simulink model "Dyn_6DoF_v2_0_r2019b"  (R2019b)
settings: Solver=ode4  StartTime=0.0  StopTime=simInit.TSIM  FixedStep=simInit.dt  MaxStep=simInit.dt  RelTol=1e-3
InitFcn:
  | close all
undefined symbols (not defined in the file): __PRM__SERIALIZED__DATA__, act, constr, DE2019, DiscIntNeverNeededParam, ENVMT, omega_rate_max, params, simInit, SubsystemReferenceBlock
libraries: simulink x16, simulink_extras x3
(part 3 of 3)

== matlab function Dyn_6DoF_v2_0_r2019b/AirborneSystem/ForcesAndTorques/aerodynamic forces FSI/Elevator Aero/Elevator_aero ==
  data: input input double; out output double size=[6,1]; DE2019 parameter; ENVMT parameter
% Copyright 2021 Delft University of Technology
%
% Licensed under the Apache License, Version 2.0 (the "License");
% you may not use this file except in compliance with the License.
% You may obtain a copy of the License at
%
%      http://www.apache.org/licenses/LICENSE-2.0
%
% Unless required by applicable law or agreed to in writing, software
% distributed under the License is distributed on an "AS IS" BASIS,
% WITHOUT WARRANTIES OR CONDITIONS OF ANY KIND, either express or implied.
% See the License for the specific language governing permissions and
% limitations under the License.

function out = simpleAero(input, DE2019, ENVMT)
%simpleAero - Elevator simple aero calculation
%
% Inputs:
%    input  - airspeed, AoA, sideslip, CL and CD
%    DE2019 - Aircraft parameters
%    ENVMT  - Environment characteristics
%
% Outputs:
%    out    - 3D forces and moments generated by the elevator
%
%
% Author: Sebastian Rapp, Ph.D., Revised by: Dylan Eijkelhof, M.Sc.
% Delft University of Technology
% email address: d.eijkelhof@tudelft.nl
% December 2019; Last revision: 19-March-2021

%-------------	BEGIN CODE	--------------
    V = input(1);
    alpha = input(2);
    beta = input(3);

    q = 0.5*ENVMT.rhos*V^2;

    F_L_el = -input(4)*q*DE2019.S_el;
    F_D_el = -input(5)*q*DE2019.S_el;

    F_x_s = F_D_el*cos(alpha)*cos(beta) - F_L_el*sin(alpha)*cos(beta);
    F_y_s = 0;
    F_z_s = F_L_el*cos(alpha);

    M_x_s = 0;
    M_y_s = F_L_el*(DE2019.x_el+DE2019.c_el*0.25);
    M_z_s = 0;

    out = [F_x_s, F_y_s, F_z_s, M_x_s, M_y_s, M_z_s]';
%-------------	END CODE	--------------
end

== matlab function Dyn_6DoF_v2_0_r2019b/AirborneSystem/FlightControlSystem/AttitudeAndRateLoop/RateLoop/Rate_Loop/Hedging/InversionRotationalDynamics1 ==
  data: nu_p_hat output; Moments input; p input; q input; r input; DE2019 parameter; nu_q_hat output; nu_r_hat output
% Copyright 2021 Delft University of Technology
%
% Licensed under the Apache License, Version 2.0 (the "License");
% you may not use this file except in compliance with the License.
% You may obtain a copy of the License at
%
%      http://www.apache.org/licenses/LICENSE-2.0
%
% Unless required by applicable law or agreed to in writing, software
% distributed under the License is distributed on an "AS IS" BASIS,
% WITHOUT WARRANTIES OR CONDITIONS OF ANY KIND, either express or implied.
% See the License for the specific language governing permissions and
% limitations under the License.

function [nu_p_hat, nu_q_hat, nu_r_hat] = hedging_rot_inv(Moments, p, q, r, DE2019)
%hedging_rot_inv - Expected error after inversion
%
% Inputs:
%    Moments   - Roll, pitch and yaw moment
%    p         - Roll rate
%    q         - Pitch rate
%    r         - Yaw rate
%    DE2019    - Aircraft parameters
%
% Outputs:
%    nu_p_hat  - Expected roll rate error
%    nu_q_hat  - Expected pitch rate error
%    nu_r_hat  - Expected yaw rate error
%
% Other m-files required:   none
% Subfunctions:             none
% MAT-files required:       none
%
% Author: Sebastian Rapp, Ph.D., Revised by: Dylan Eijkelhof, M.Sc.
% Delft University of Technology
% email address: d.eijkelhof@tudelft.nl
% December 2019; Last revision: 19-March-2021

%------------- BEGIN CODE --------------
 
L = Moments(1); 
M = Moments(2); 
N = Moments(3); 

Jx =  DE2019.J(1,1); 
Jy =  DE2019.J(2,2); 
Jz =  DE2019.J(3,3); 
 
nu_p_hat = 1/Jx * (L - q * r * Jz +  q * r * Jy ); 
nu_q_hat = 1/Jy *(M - r * p * Jx + r * p * Jz  );
nu_r_hat = 1/Jz * (N - p * q * Jy + p * q * Jx ); 

%------------- END CODE --------------
end

== matlab function Dyn_6DoF_v2_0_r2019b/AirborneSystem/FlightControlSystem/AttitudeAndRateLoop/RateLoop/Rate_Loop/InversionRotationalDynamics ==
  data: omega_OB_B input; M_des output; nu_NDI input; DE2019 parameter
% Copyright 2021 Delft University of Technology
%
% Licensed under the Apache License, Version 2.0 (the "License");
% you may not use this file except in compliance with the License.
% You may obtain a copy of the License at
%
%      http://www.apache.org/licenses/LICENSE-2.0
%
% Unless required by applicable law or agreed to in writing, software
% distributed under the License is distributed on an "AS IS" BASIS,
% WITHOUT WARRANTIES OR CONDITIONS OF ANY KIND, either express or implied.
% See the License for the specific language governing permissions and
% limitations under the License.

function M_des  = Rate_inv(omega_OB_B,nu_NDI,  DE2019)
%Rate_inv - Determine desired moments
%
% Inputs:
%    omega_OB_B - Commanded roll, pitch and yaw rates
%    nu_NDI     - Roll, pitch and yaw rate error incl. controller gains
%    DE2019     - Aircraft parameters
%
% Outputs:
%    M_des  - Expected roll rate error
%
% Other m-files required:   none
% Subfunctions:             none
% MAT-files required:       none
%
% Author: Sebastian Rapp, Ph.D., Revised by: Dylan Eijkelhof, M.Sc.
% Delft University of Technology
% email address: d.eijkelhof@tudelft.nl
% December 2019; Last revision: 19-March-2021

%------------- BEGIN CODE --------------

p = omega_OB_B(1); 
q = omega_OB_B(2); 
r = omega_OB_B(3); 

nu_p = nu_NDI(1); 
nu_q = nu_NDI(2); 
nu_r = nu_NDI(3); 
 
Jx = DE2019.J(1,1); 
Jy = DE2019.J(2,2); 
Jz = DE2019.J(3,3);

Lc = Jx * nu_p + q * r * Jz  - q * r * Jy; 
Mc = Jy * nu_q + r * p * Jx - r * p * Jz;
Nc = Jz * nu_r + p * q * Jy - p * q * Jx; 

M_des = [Lc; Mc; Nc];

%------------- END CODE --------------
end

== matlab function Dyn_6DoF_v2_0_r2019b/AirborneSystem/ForcesAndTorques/aerodynamic forces FSI/Rudder Aero/Rudder_aero ==
  data: input input double; out output double size=[6,1]; DE2019 parameter; ENVMT parameter
% Copyright 2021 Delft University of Technology
%
% Licensed under the Apache License, Version 2.0 (the "License");
% you may not use this file except in compliance with the License.
% You may obtain a copy of the License at
%
%      http://www.apache.org/licenses/LICENSE-2.0
%
% Unless required by applicable law or agreed to in writing, software
% distributed under the License is distributed on an "AS IS" BASIS,
% WITHOUT WARRANTIES OR CONDITIONS OF ANY KIND, either express or implied.
% See the License for the specific language governing permissions and
% limitations under the License.

function out = simpleAero(input, DE2019, ENVMT)
%simpleAero - Rudder simple aero calculation
%
% Inputs:
%    input  - airspeed, AoA, sideslip, CL and CD
%    DE2019 - Aircraft parameters
%    ENVMT  - Environment characteristics
%
% Outputs:
%    out    - 3D forces and moments generated by the rudder
%
%
% Author: Sebastian Rapp, Ph.D., Revised by: Dylan Eijkelhof, M.Sc.
% Delft University of Technology
% email address: d.eijkelhof@tudelft.nl
% December 2019; Last revision: 19-March-2021

%-------------	BEGIN CODE	--------------
    V = input(1);
    alpha = input(2);
    beta = input(3);

    q = 0.5*ENVMT.rhos*V^2;
   
    F_L_vs = 2*input(4)*q*DE2019.S_vs;
    F_D_vs = -2*input(5)*q*DE2019.S_vs;

    F_x_s = F_D_vs*cos(alpha)*cos(beta);
    F_y_s = -F_L_vs*cos(beta);
    F_z_s = 0;

    M_x_s = F_L_vs*(DE2019.b_vs*0.5);
    M_y_s = 0;
    M_z_s = F_L_vs*(DE2019.x_vs+DE2019.c_vs*0.25);

    out = [F_x_s, F_y_s, F_z_s, M_x_s, M_y_s, M_z_s]';
%-------------	END CODE	--------------  
end

== matlab function Dyn_6DoF_v2_0_r2019b/RequirementModelsAndLogging/Power_convergence/MATLAB Function ==
  settings: updateMethod=DISCRETE  sampleTime=simInit.Ts_power_conv_check
  data: flag output; m_new output; p_sum output; cnt output; flag input; m_old input; p_sum input; cnt input; u input; flightMode input; e_new output; e_old input; cnt_max_mat input; cnt_max_mat output; cycles_cnt input; cycles_cnt output
% Copyright 2021 Delft University of Technology
%
% Licensed under the Apache License, Version 2.0 (the "License");
% you may not use this file except in compliance with the License.
% You may obtain a copy of the License at
%
%      http://www.apache.org/licenses/LICENSE-2.0
%
% Unless required by applicable law or agreed to in writing, software
% distributed under the License is distributed on an "AS IS" BASIS,
% WITHOUT WARRANTIES OR CONDITIONS OF ANY KIND, either express or implied.
% See the License for the specific language governing permissions and
% limitations under the License.

function [flag, m_new, p_sum, cnt, e_new, cnt_max_mat,cycles_cnt] = fcn(flag, m_old, p_sum, cnt, u, flightMode, e_old,cnt_max_mat,cycles_cnt)
% function [flag, m_new, p_sum, cnt, e_new, cnt_max_mat,cycles_cnt] = fcn(flag, m_old, p_sum, cnt, u, flightMode, e_old,cnt_max_mat,cycles_cnt, cnt_extra)
%y = [u;old(1:end-1)];
% if cnt > nmax
%     new_mean = mean(y);
%     cnt = 0;
% end
p_sum = p_sum + u;
cnt = cnt + 1;

if flightMode == 5 && flag
    cnt_max_mat = cnt; 
    m_new = p_sum/cnt;
    cnt  = 0;
    cycles_cnt = cycles_cnt + 1;
    p_sum = 0;
    flag = 0;
    e_new = abs( m_new - m_old );
elseif flightMode == 6
%     if cnt_extra == 0 || cycles_cnt == 0
%         cycles_cnt = cycles_cnt + 1;
%     end
    flag = 1;
    m_new = m_old;
    e_new = e_old;
else
    flag = 0;
    m_new = m_old;
    e_new = e_old;
end

% m_new = m_old + (u-old(nmax))/nmax;
